simulink model "amortiguadorVehiculoBueno"  (R2022b)
settings: Solver=VariableStepAuto  StartTime=0.0  StopTime=10  MaxStep=1  RelTol=1e-3
values from neighbouring files (symbols this model uses):
  b1 = 1000    [Amortiguador1.m]    (also in DatosAmortiguadores.m)
  f = 0    [Amortiguador1.m]    (also in DatosAmortiguadores.m)
  k1 = 16182    [Amortiguador1.m]    (also in DatosAmortiguadores.m)
  k2 = 19000    [Amortiguador1.m]    (also in DatosAmortiguadores.m)
  m1 = 290    [Amortiguador1.m]    (also in DatosAmortiguadores.m)
  m2 = 59    [Amortiguador1.m]    (also in DatosAmortiguadores.m)
settings Model: Creator=bryan  LastModifiedBy=perez

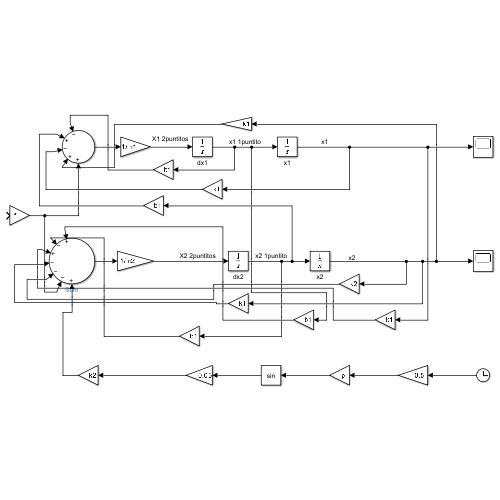
[thumbnail: Simulink's stored preview of the top-level diagram]
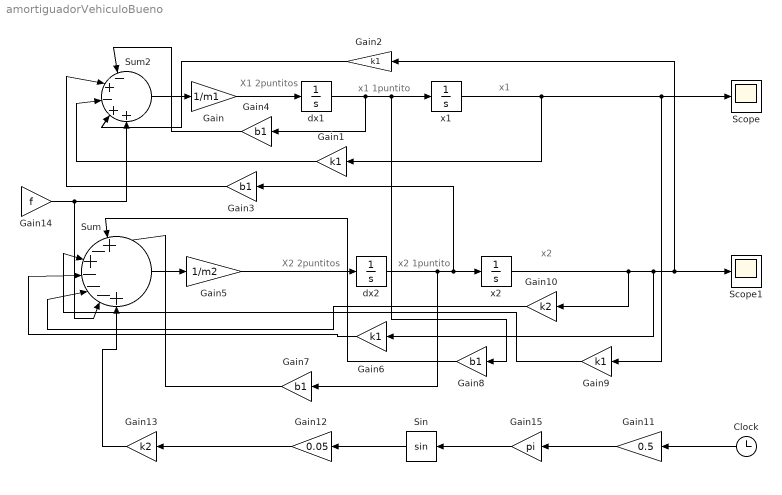
== system amortiguadorVehiculoBueno ==
  note: x1
  note: x2
  note: x1 1puntito
  note: X2 2puntitos
  note: X1 2puntitos
  note: x2 1puntito
  Clock : Clock
  Gain : Gain  Gain=1/m1
  Gain{1..2,6,9} (4 alike) : Gain  Gain=k1
  Gain10 : Gain  Gain=k2
  Gain11 : Gain  Gain=0.5
  Gain12 : Gain  Gain=0.05
  Gain13 : Gain  Gain=k2
  Gain14 : Gain  Gain=f
  Gain15 : Gain  Gain=pi
  Gain{3..4,7..8} (4 alike) : Gain  Gain=b1
  Gain5 : Gain  Gain=1/m2
  Scope : Scope
  Scope1 : Scope
  Sin : Trigonometry
  Sum : Sum  Inputs=|+|-|+|-|-|-|+
  Sum2 : Sum  Inputs=|-|+|-|+|+
  dx1 : Integrator
  dx2 : Integrator
  x1 : Integrator
  x2 : Integrator
  wires:
  dx1/1 -> Gain4/1, x1/1, Gain8/1
  x1/1 -> Scope/1, Gain9/1, Gain1/1
  Gain/1 -> dx1/1
  Gain4/1 -> Sum2/1
  Gain1/1 -> Sum2/3
  Gain3/1 -> Sum2/2
  Gain2/1 -> Sum2/4
  dx2/1 -> Gain7/1, Gain3/1, x2/1
  Gain5/1 -> dx2/1
  Gain10/1 -> Sum/5
  Gain6/1 -> Sum/4
  Gain8/1 -> Sum/1
  Gain7/1 -> Sum/2
  Gain9/1 -> Sum/3
  x2/1 -> Gain10/1, Gain6/1, Scope1/1, Gain2/1
  Gain11/1 -> Gain15/1
  Sin/1 -> Gain12/1
  Gain12/1 -> Gain13/1
  Gain13/1 -> Sum/7
  Gain14/1 -> Sum2/5, Sum/6
  Gain15/1 -> Sin/1
  Clock/1 -> Gain11/1
  Sum2/1 -> Gain/1
  Sum/1 -> Gain5/1
